simulink model "MultiVehicleModel"  (R2014a)
settings: Solver=ode1  StartTime=0.0  StopTime=inf  FixedStep=simPars.SampleTime  RelTol=1e-3
undefined symbols (not defined in the file or in its folder): DiscIntNeverNeededParam, Earth, Env, eul_0, FWFleet, GVFleet, m, RCFleet, s, WGS84
undefined symbols (not defined in the file): simPars
libraries: simulink x26, aerolibtransform2 x7, instrumentlib x6, Actuator_Lib x5, aerolib6dofsys x4, etargetslib x3, aerolibasang x3, aerolibconvert2 x2, aerolibutil x1, aerolibatmos2 x1, aerolibobsolete x1, aerolibgravity2 x1
(part 2 of 4)

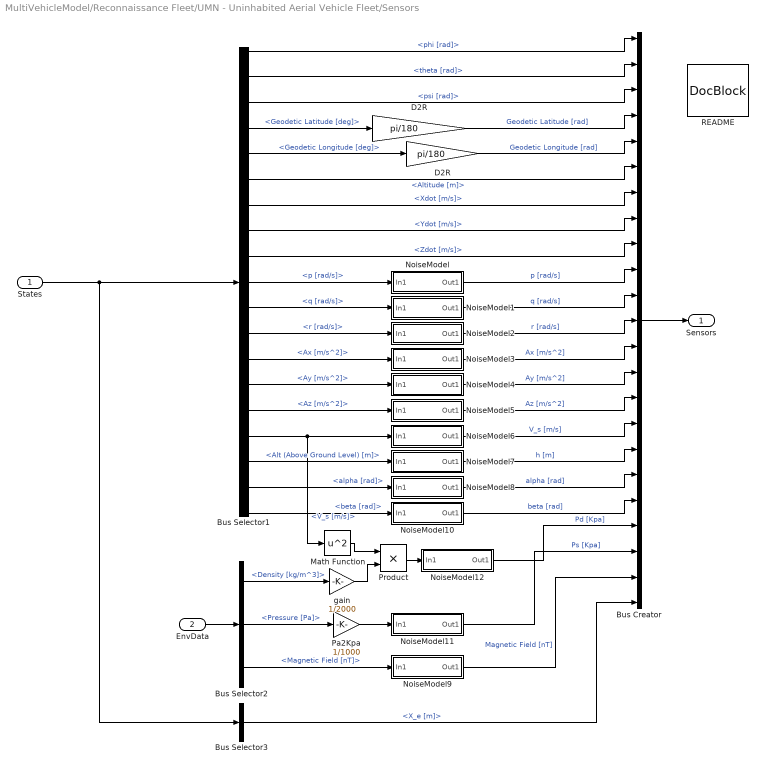
== system MultiVehicleModel/Reconnaissance Fleet/UMN - Uninhabited Aerial Vehicle Fleet/Sensors ==
  States : Inport
  EnvData : Inport  Port=2
  Bus Creator : BusCreator  Inputs=23
  Bus Selector1 : BusSelector  OutputSignals=Euler [rad].phi [rad],Euler [rad].theta [rad],Euler [rad].psi [rad],Nav.Geodetic Latitude [deg],Nav.Geodetic Longitude [deg],Nav.Altitude [m],V_e [m/s].Xdot [m/s],V_e [m/s].Ydot [m/s],V_e [m/s].Zdot [m/s],AngVel [rad/s].p [rad/s],AngVel [rad/s].q [rad/s],AngVel [rad/s].r [rad/s],Accels [m/s^2].Ax [m/s^2],Accels [m/s^2].Ay [m/s^2],Accels [m/s^2].Az [m/s^2],WindAxesParam.V_s [m/s],Nav.Alt (Above Ground Level) [m],WindAxesParam.alpha [rad],WindAxesParam.beta [rad]
  Bus Selector2 : BusSelector  OutputSignals=Density [kg/m^3],Pressure [Pa],Magnetic Field [nT]
  Bus Selector3 : BusSelector  OutputSignals=X_e [m]
  D2R : Gain  Gain=pi/180  SampleTime=SampleTime
  "D2R " : Gain  Gain=pi/180  SampleTime=SampleTime
  Math Function : Math  Operator=square  SaturateOnIntegerOverflow=on
  NoiseModel : Subsystem  mask(Sensor Model){noise_on=AC.Sensors.NoiseOn, sigma=AC.Sensors.IMU.p_noise, seed=878230, bias=AC.Sensors.IMU.p_bias, scf=AC.Sensors.IMU.p_scf, timestep=SampleTime}
      mask prompts: noise_on "on/off"; scf "scale factor:"
      mask help:
      | Add bias, scale factor, and white noise to a signal
      |
      | - 'on/off': 1 = noise on, 0 = noise off.
      | - 'sigma' : Standard deviation of white noise.
      | - 'seed'  : Random number seed.
      | - 'bias'  : Constant mean value offset of white noise.
      | - 'scale factor' : Scale factor applied to original signal.
      | - 'Timestep': Time step of the simulation
      mask Display: disp('bias/scf/noise')
  NoiseModel1 : Subsystem  mask(Sensor Model){noise_on=AC.Sensors.NoiseOn, sigma=AC.Sensors.IMU.q_noise, seed=878231, bias=AC.Sensors.IMU.q_bias, scf=AC.Sensors.IMU.q_scf, timestep=SampleTime}
      mask prompts: noise_on "on/off"; scf "scale factor:"
      mask help:
      | Add bias, scale factor, and white noise to a signal
      |
      | - 'on/off': 1 = noise on, 0 = noise off.
      | - 'sigma' : Standard deviation of white noise.
      | - 'seed'  : Random number seed.
      | - 'bias'  : Constant mean value offset of white noise.
      | - 'scale factor' : Scale factor applied to original signal.
      | - 'Timestep': Time step of the simulation
      mask Display: disp('bias/scf/noise')
  NoiseModel10 : Subsystem  mask(Sensor Model){noise_on=AC.Sensors.NoiseOn, sigma=AC.Sensors.AirData.beta_noise, seed=87828, bias=AC.Sensors.AirData.beta_bias, scf=AC.Sensors.AirData.beta_scf, timestep=SampleTime}
      mask prompts: noise_on "on/off"; scf "scale factor:"
      mask help:
      | Add bias, scale factor, and white noise to a signal
      |
      | - 'on/off': 1 = noise on, 0 = noise off.
      | - 'sigma' : Standard deviation of white noise.
      | - 'seed'  : Random number seed.
      | - 'bias'  : Constant mean value offset of white noise.
      | - 'scale factor' : Scale factor applied to original signal.
      | - 'Timestep': Time step of the simulation
      mask Display: disp('bias/scf/noise')
  NoiseModel11 : Subsystem  mask(Sensor Model){noise_on=AC.Sensors.NoiseOn, sigma=AC.Sensors.AirData.Ps_noise, seed=8782378, bias=AC.Sensors.AirData.Ps_bias, scf=AC.Sensors.AirData.Ps_scf, timestep=SampleTime}
      mask prompts: noise_on "on/off"; scf "scale factor:"
      mask help:
      | Add bias, scale factor, and white noise to a signal
      |
      | - 'on/off': 1 = noise on, 0 = noise off.
      | - 'sigma' : Standard deviation of white noise.
      | - 'seed'  : Random number seed.
      | - 'bias'  : Constant mean value offset of white noise.
      | - 'scale factor' : Scale factor applied to original signal.
      | - 'Timestep': Time step of the simulation
      mask Display: disp('bias/scf/noise')
  NoiseModel12 : Subsystem  mask(Sensor Model){noise_on=AC.Sensors.NoiseOn, sigma=AC.Sensors.AirData.Pd_noise, seed=87823, bias=AC.Sensors.AirData.Pd_bias, scf=AC.Sensors.AirData.Pd_scf, timestep=SampleTime}
      mask prompts: noise_on "on/off"; scf "scale factor:"
      mask help:
      | Add bias, scale factor, and white noise to a signal
      |
      | - 'on/off': 1 = noise on, 0 = noise off.
      | - 'sigma' : Standard deviation of white noise.
      | - 'seed'  : Random number seed.
      | - 'bias'  : Constant mean value offset of white noise.
      | - 'scale factor' : Scale factor applied to original signal.
      | - 'Timestep': Time step of the simulation
      mask Display: disp('bias/scf/noise')
  NoiseModel2 : Subsystem  mask(Sensor Model){noise_on=AC.Sensors.NoiseOn, sigma=AC.Sensors.IMU.r_noise, seed=878232, bias=AC.Sensors.IMU.r_bias, scf=AC.Sensors.IMU.r_scf, timestep=SampleTime}
      mask prompts: noise_on "on/off"; scf "scale factor:"
      mask help:
      | Add bias, scale factor, and white noise to a signal
      |
      | - 'on/off': 1 = noise on, 0 = noise off.
      | - 'sigma' : Standard deviation of white noise.
      | - 'seed'  : Random number seed.
      | - 'bias'  : Constant mean value offset of white noise.
      | - 'scale factor' : Scale factor applied to original signal.
      | - 'Timestep': Time step of the simulation
      mask Display: disp('bias/scf/noise')
  NoiseModel3 : Subsystem  mask(Sensor Model){noise_on=AC.Sensors.NoiseOn, sigma=AC.Sensors.IMU.ax_noise, seed=878233, bias=AC.Sensors.IMU.ax_bias, scf=AC.Sensors.IMU.ax_scf, timestep=SampleTime}
      mask prompts: noise_on "on/off"; scf "scale factor:"
      mask help:
      | Add bias, scale factor, and white noise to a signal
      |
      | - 'on/off': 1 = noise on, 0 = noise off.
      | - 'sigma' : Standard deviation of white noise.
      | - 'seed'  : Random number seed.
      | - 'bias'  : Constant mean value offset of white noise.
      | - 'scale factor' : Scale factor applied to original signal.
      | - 'Timestep': Time step of the simulation
      mask Display: disp('bias/scf/noise')
  NoiseModel4 : Subsystem  mask(Sensor Model){noise_on=AC.Sensors.NoiseOn, sigma=AC.Sensors.IMU.ay_noise, seed=878234, bias=AC.Sensors.IMU.ay_bias, scf=AC.Sensors.IMU.ay_scf, timestep=SampleTime}
      mask prompts: noise_on "on/off"; scf "scale factor:"
      mask help:
      | Add bias, scale factor, and white noise to a signal
      |
      | - 'on/off': 1 = noise on, 0 = noise off.
      | - 'sigma' : Standard deviation of white noise.
      | - 'seed'  : Random number seed.
      | - 'bias'  : Constant mean value offset of white noise.
      | - 'scale factor' : Scale factor applied to original signal.
      | - 'Timestep': Time step of the simulation
      mask Display: disp('bias/scf/noise')
  NoiseModel5 : Subsystem  mask(Sensor Model){noise_on=AC.Sensors.NoiseOn, sigma=AC.Sensors.IMU.az_noise, seed=878235, bias=AC.Sensors.IMU.az_bias, scf=AC.Sensors.IMU.az_scf, timestep=SampleTime}
      mask prompts: noise_on "on/off"; scf "scale factor:"
      mask help:
      | Add bias, scale factor, and white noise to a signal
      |
      | - 'on/off': 1 = noise on, 0 = noise off.
      | - 'sigma' : Standard deviation of white noise.
      | - 'seed'  : Random number seed.
      | - 'bias'  : Constant mean value offset of white noise.
      | - 'scale factor' : Scale factor applied to original signal.
      | - 'Timestep': Time step of the simulation
      mask Display: disp('bias/scf/noise')
  NoiseModel6 : Subsystem  mask(Sensor Model){noise_on=AC.Sensors.NoiseOn, sigma=AC.Sensors.AirData.ias_noise, seed=878236, bias=AC.Sensors.AirData.ias_bias, scf=AC.Sensors.AirData.ias_scf, timestep=SampleTime}
      mask prompts: noise_on "on/off"; scf "scale factor:"
      mask help:
      | Add bias, scale factor, and white noise to a signal
      |
      | - 'on/off': 1 = noise on, 0 = noise off.
      | - 'sigma' : Standard deviation of white noise.
      | - 'seed'  : Random number seed.
      | - 'bias'  : Constant mean value offset of white noise.
      | - 'scale factor' : Scale factor applied to original signal.
      | - 'Timestep': Time step of the simulation
      mask Display: disp('bias/scf/noise')
  NoiseModel7 : Subsystem  mask(Sensor Model){noise_on=AC.Sensors.NoiseOn, sigma=AC.Sensors.AirData.h_noise, seed=87828, bias=AC.Sensors.AirData.h_bias, scf=AC.Sensors.AirData.h_scf, timestep=SampleTime}
      mask prompts: noise_on "on/off"; scf "scale factor:"
      mask help:
      | Add bias, scale factor, and white noise to a signal
      |
      | - 'on/off': 1 = noise on, 0 = noise off.
      | - 'sigma' : Standard deviation of white noise.
      | - 'seed'  : Random number seed.
      | - 'bias'  : Constant mean value offset of white noise.
      | - 'scale factor' : Scale factor applied to original signal.
      | - 'Timestep': Time step of the simulation
      mask Display: disp('bias/scf/noise')
  NoiseModel8 : Subsystem  mask(Sensor Model){noise_on=AC.Sensors.NoiseOn, sigma=AC.Sensors.AirData.alpha_noise, seed=87828, bias=AC.Sensors.AirData.alpha_bias, scf=AC.Sensors.AirData.alpha_scf, timestep=SampleTime}
      mask prompts: noise_on "on/off"; scf "scale factor:"
      mask help:
      | Add bias, scale factor, and white noise to a signal
      |
      | - 'on/off': 1 = noise on, 0 = noise off.
      | - 'sigma' : Standard deviation of white noise.
      | - 'seed'  : Random number seed.
      | - 'bias'  : Constant mean value offset of white noise.
      | - 'scale factor' : Scale factor applied to original signal.
      | - 'Timestep': Time step of the simulation
      mask Display: disp('bias/scf/noise')
  NoiseModel9 : Subsystem  mask(Sensor Model){noise_on=AC.Sensors.NoiseOn, sigma=[AC.Sensors.IMU.hx_noise, AC.Sensors.IMU.hy_noise,AC.Sensors.IMU.hz_noise], seed=878237, bias=[AC.Sensors.IMU.hx_bias, AC.Sensors.IMU.hy_bias, AC.Sensors.IMU.hz_bias], scf=[AC.Sensors.IMU.hx_scf, AC.Sensors.IMU.hy_scf, AC.Sensors.IMU.hz_scf], timestep=SampleTime}
      mask prompts: noise_on "on/off"; scf "scale factor:"
      mask help:
      | Add bias, scale factor, and white noise to a signal
      |
      | - 'on/off': 1 = noise on, 0 = noise off.
      | - 'sigma' : Standard deviation of white noise.
      | - 'seed'  : Random number seed.
      | - 'bias'  : Constant mean value offset of white noise.
      | - 'scale factor' : Scale factor applied to original signal.
      | - 'Timestep': Time step of the simulation
      mask Display: disp('bias/scf/noise')
  Pa2Kpa : Gain  Gain=1/1000
  Product : Product  RndMeth=Zero
  README : simulink/Model-Wide Utilities/DocBlock  DocumentType=Text
      content=|
      | Sensors
      |
      | This block implements sensor models on selected signals. A generic block
      | is used that applies a bias, scale factor, and band limited white noise to
      | a given signal. The parameters for each block are stored in the aircraft
      | configuration data structure (AC):
      |
      | >> AC.Sensors
      |
      | ans =
      |
      |     NoiseOn: 1
      |         IMU: [1x1 struct]
      |     AirData: [1x1 struct]
      |
      | Note the "NoiseOn" boolean flag- by setting this flag to zero, the sensor
      | model will be disabled.
      |
      | Currently, the bias and scale factor errors are not used; only white noise
      | is applied.
  gain : Gain  Gain=1/2000
  Sensors : Outport
  wires:
  Bus Selector1/15 -> NoiseModel5/1(In1)  "<Az [m/s^2]>"
  Bus Selector1/14 -> NoiseModel4/1(In1)  "<Ay [m/s^2]>"
  Bus Selector1/13 -> NoiseModel3/1(In1)  "<Ax [m/s^2]>"
  Bus Selector1/12 -> NoiseModel2/1(In1)  "<r [rad/s]>"
  Bus Selector1/11 -> NoiseModel1/1(In1)  "<q [rad/s]>"
  Bus Selector1/10 -> NoiseModel/1(In1)  "<p [rad/s]>"
  States/1 -> Bus Selector3/1, Bus Selector1/1
  Bus Selector1/16 -> NoiseModel6/1(In1), Math Function/1  "<V_s [m/s]>"
  Bus Selector2/3 -> NoiseModel9/1(In1)  "<Magnetic Field [nT]>"
  Bus Selector1/17 -> NoiseModel7/1(In1)  "<Alt (Above Ground Level) [m]>"
  EnvData/1 -> Bus Selector2/1
  Bus Selector1/18 -> NoiseModel8/1(In1)  "<alpha [rad]>"
  Bus Selector1/19 -> NoiseModel10/1(In1)  "<beta [rad]>"
  Bus Selector2/2 -> Pa2Kpa/1  "<Pressure [Pa]>"
  Pa2Kpa/1 -> NoiseModel11/1(In1)
  Bus Selector2/1 -> gain/1  "<Density [kg/m^3]>"
  Math Function/1 -> Product/1
  gain/1 -> Product/2
  Product/1 -> NoiseModel12/1(In1)
  Bus Creator/1 -> Sensors/1
  Bus Selector1/1 -> Bus Creator/1  "<phi [rad]>"
  Bus Selector1/2 -> Bus Creator/2  "<theta [rad]>"
  Bus Selector1/3 -> Bus Creator/3  "<psi [rad]>"
  Bus Selector1/4 -> D2R/1  "<Geodetic Latitude [deg]>"
  Bus Selector1/5 -> "D2R "/1  "<Geodetic Longitude [deg]>"
  Bus Selector1/6 -> Bus Creator/6  "<Altitude [m]>"
  Bus Selector1/7 -> Bus Creator/7  "<Xdot [m/s]>"
  Bus Selector1/8 -> Bus Creator/8  "<Ydot [m/s]>"
  Bus Selector1/9 -> Bus Creator/9  "<Zdot [m/s]>"
  NoiseModel/1(Out1) -> Bus Creator/10  "p [rad/s]"
  NoiseModel1/1(Out1) -> Bus Creator/11  "q [rad/s]"
  NoiseModel2/1(Out1) -> Bus Creator/12  "r [rad/s]"
  NoiseModel3/1(Out1) -> Bus Creator/13  "Ax [m/s^2]"
  NoiseModel4/1(Out1) -> Bus Creator/14  "Ay [m/s^2]"
  NoiseModel5/1(Out1) -> Bus Creator/15  "Az [m/s^2]"
  NoiseModel6/1(Out1) -> Bus Creator/16  "V_s [m/s]"
  NoiseModel7/1(Out1) -> Bus Creator/17  "h [m]"
  NoiseModel8/1(Out1) -> Bus Creator/18  "alpha [rad]"
  NoiseModel10/1(Out1) -> Bus Creator/19  "beta [rad]"
  NoiseModel12/1(Out1) -> Bus Creator/20  "Pd [Kpa]"
  NoiseModel11/1(Out1) -> Bus Creator/21  "Ps [Kpa]"
  NoiseModel9/1(Out1) -> Bus Creator/22  "Magnetic Field [nT]"
  D2R/1 -> Bus Creator/4  "Geodetic Latitude [rad]"
  "D2R "/1 -> Bus Creator/5  "Geodetic Longitude [rad]"
  Bus Selector3/1 -> Bus Creator/23  "<X_e [m]>"

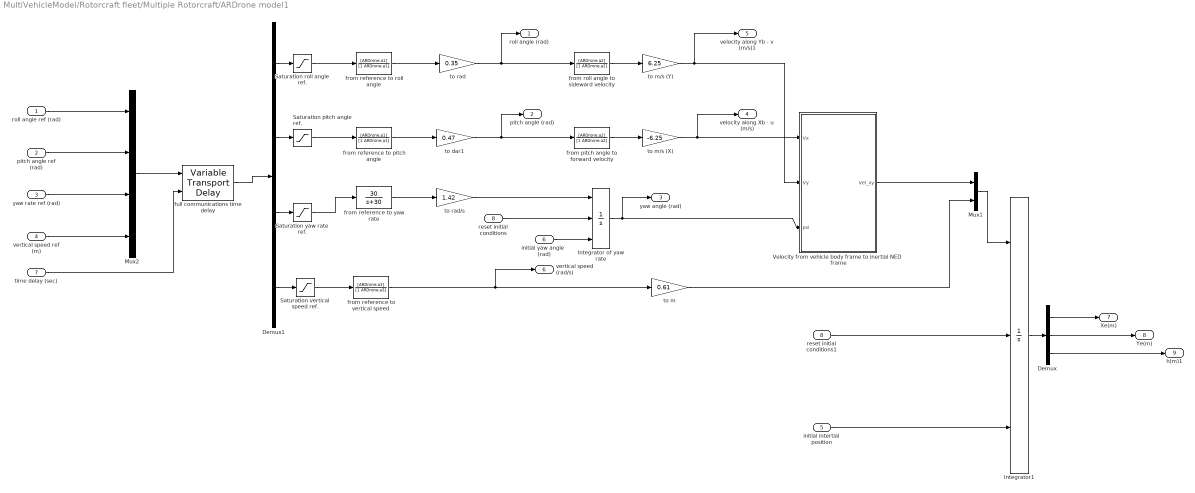
== system MultiVehicleModel/Rotorcraft fleet/Multiple Rotorcraft/ARDrone model1 ==
  roll angle ref (rad) : Inport
  pitch angle ref (rad) : Inport  Port=2
  yaw rate ref (rad) : Inport  Port=3
  vertical speed ref (m) : Inport  Port=4
  initial intertial position : Inport  Port=5
  initial yaw angle  (rad) : Inport  Port=6
  time delay (sec) : Inport  Port=7
  reset initial conditions : Inport  Port=8
  Demux : Demux  Outputs=3
  Demux1 : Demux
  Integrator of yaw rate : Integrator  ExternalReset=rising  InitialConditionSource=external
  Integrator1 : Integrator  ExternalReset=rising  InitialConditionSource=external
  Mux1 : Mux  Inputs=2
  Mux2 : Mux
  Saturation pitch angle ref. : Saturate  UpperLimit=ARDrone.MAX_ANGLE_REF  LowerLimit=ARDrone.MIN_ANGLE_REF
  Saturation roll angle ref. : Saturate  UpperLimit=ARDrone.MAX_ANGLE_REF  LowerLimit=ARDrone.MIN_ANGLE_REF
  Saturation vertical speed ref. : Saturate  UpperLimit=ARDrone.MAX_VERTICAL_SPEED  LowerLimit=ARDrone.MIN_VERTICAL_SPEED
  Saturation yaw rate ref. : Saturate  UpperLimit=ARDrone.MAX_YAW_RATE_REF  LowerLimit=ARDrone.MIN_YAW_RATE_REF
  Velocity from vehicle body frame to inertial NED  frame : MATLAB Function  TreatAsAtomicUnit=on
  from pitch angle to forward velocity : TransferFcn  Numerator=[ARDrone.a2]  Denominator=[1 ARDrone.a2]
  from reference to pitch angle : TransferFcn  Numerator=[ARDrone.a1]  Denominator=[1 ARDrone.a1]
  from reference to roll angle : TransferFcn  Numerator=[ARDrone.a1]  Denominator=[1 ARDrone.a1]
  from reference to vertical speed : TransferFcn  Numerator=[ARDrone.a3]  Denominator=[1 ARDrone.a3]
  from reference to yaw rate : TransferFcn  Numerator=[30]  Denominator=[1 30]
  from roll angle to sideward velocity : TransferFcn  Numerator=[ARDrone.a2]  Denominator=[1 ARDrone.a2]
  full communications time delay : VariableTransportDelay  MaximumDelay=10  InitialOutput=[0 0 0 0]
  reset initial conditions1 : InportShadow  Port=8
  to dar1 : Gain  Gain=0.47
  to m : Gain  Gain=0.61
  to m/s (X) : Gain  Gain=-6.25
  to m/s (Y) : Gain  Gain=6.25
  to rad : Gain  Gain=0.35
  to rad/s : Gain  Gain=1.42
  roll angle (rad) : Outport
  pitch angle (rad) : Outport  Port=2
  yaw angle (rad) : Outport  Port=3
  velocity along Xb - u (m/s) : Outport  Port=4
  velocity along Yb - v (m/s)1 : Outport  Port=5
  vertical speed (rad/s) : Outport  Port=6
  Xe(m) : Outport  Port=7
  Ye(m) : Outport  Port=8
  h(m)1 : Outport  Port=9
  wires:
  from reference to pitch angle/1 -> to dar1/1
  from reference to roll angle/1 -> to rad/1
  Saturation roll angle ref./1 -> from reference to roll angle/1
  from reference to yaw rate/1 -> to rad/s/1
  Saturation vertical speed ref./1 -> from reference to vertical speed/1
  from pitch angle to forward velocity/1 -> to m/s (X)/1
  from roll angle to sideward velocity/1 -> to m/s (Y)/1
  Demux1/2 -> Saturation pitch angle ref./1
  Demux1/3 -> Saturation yaw rate ref./1
  Integrator of yaw rate/1 -> Velocity from vehicle body frame to inertial NED  frame/3(psi), yaw angle (rad)/1
  Mux1/1 -> Integrator1/1
  Velocity from vehicle body frame to inertial NED  frame/1(Vel_xy) -> Mux1/1
  from reference to vertical speed/1 -> vertical speed (rad/s)/1, to m/1
  Integrator1/1 -> Demux/1
  Demux1/1 -> Saturation roll angle ref./1
  to rad/1 -> from roll angle to sideward velocity/1, roll angle (rad)/1
  to dar1/1 -> from pitch angle to forward velocity/1, pitch angle (rad)/1
  Demux/3 -> h(m)1/1
  Demux/2 -> Ye(m)/1
  Demux/1 -> Xe(m)/1
  time delay (sec)/1 -> full communications time delay/2
  Mux2/1 -> full communications time delay/1
  full communications time delay/1 -> Demux1/1
  roll angle ref (rad)/1 -> Mux2/1
  pitch angle ref (rad)/1 -> Mux2/2
  yaw rate ref (rad)/1 -> Mux2/3
  vertical speed ref (m)/1 -> Mux2/4
  Demux1/4 -> Saturation vertical speed ref./1
  initial intertial position/1 -> Integrator1/3
  initial yaw angle  (rad)/1 -> Integrator of yaw rate/3
  reset initial conditions/1 -> Integrator of yaw rate/2
  reset initial conditions1/1 -> Integrator1/2
  to rad/s/1 -> Integrator of yaw rate/1
  to m/s (X)/1 -> Velocity from vehicle body frame to inertial NED  frame/1(Vx), velocity along Xb - u (m/s)/1
  to m/1 -> Mux1/2
  Saturation yaw rate ref./1 -> from reference to yaw rate/1
  to m/s (Y)/1 -> Velocity from vehicle body frame to inertial NED  frame/2(Vy), velocity along Yb - v (m/s)1/1
  Saturation pitch angle ref./1 -> from reference to pitch angle/1

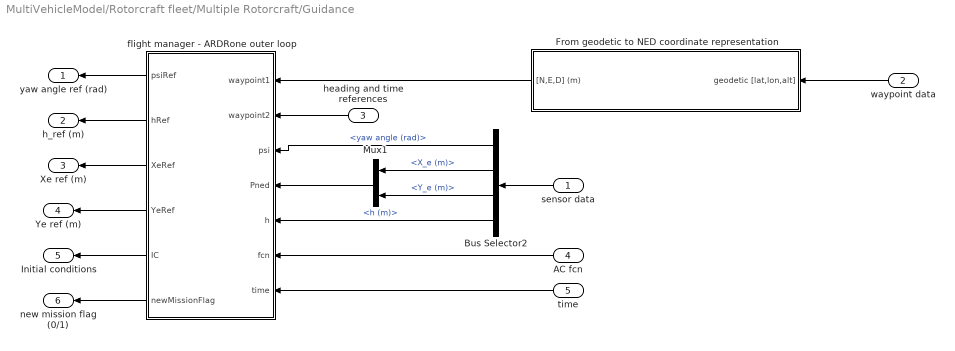
== system MultiVehicleModel/Rotorcraft fleet/Multiple Rotorcraft/Guidance  ==
  sensor data : Inport
  waypoint data : Inport  Port=2
  heading and time references : Inport  Port=3
  AC fcn : Inport  Port=4
  time : Inport  Port=5
  Bus Selector2 : BusSelector  OutputSignals=yaw angle (rad),X_e (m),Y_e (m),h (m)
  From geodetic to NED coordinate representation : Subsystem  TreatAsAtomicUnit=on
  Mux1 : Mux  Inputs=2
  flight manager - ARDRone outer loop : MATLAB Function  TreatAsAtomicUnit=on
  yaw angle ref (rad) : Outport
  h_ref (m) : Outport  Port=2
  Xe ref (m) : Outport  Port=3
  Ye ref (m) : Outport  Port=4
  Initial conditions : Outport  Port=5
  new mission flag (0/1) : Outport  Port=6
  wires:
  Bus Selector2/2 -> Mux1/1  "<X_e (m)>"
  Bus Selector2/3 -> Mux1/2  "<Y_e (m)>"
  sensor data/1 -> Bus Selector2/1
  Bus Selector2/1 -> flight manager - ARDRone outer loop/3(psi)  "<yaw angle (rad)>"
  Mux1/1 -> flight manager - ARDRone outer loop/4(Pned)
  waypoint data/1 -> From geodetic to NED coordinate representation/1(geodetic [lat,lon,alt])
  AC fcn/1 -> flight manager - ARDRone outer loop/6(fcn)
  flight manager - ARDRone outer loop/2(hRef) -> h_ref (m)/1
  flight manager - ARDRone outer loop/1(psiRef) -> yaw angle ref (rad)/1
  flight manager - ARDRone outer loop/3(XeRef) -> Xe ref (m)/1
  flight manager - ARDRone outer loop/4(YeRef) -> Ye ref (m)/1
  Bus Selector2/4 -> flight manager - ARDRone outer loop/5(h)  "<h (m)>"
  time/1 -> flight manager - ARDRone outer loop/7(time)
  From geodetic to NED coordinate representation/1("[N,E,D] (m)") -> flight manager - ARDRone outer loop/1(waypoint1)
  heading and time references/1 -> flight manager - ARDRone outer loop/2(waypoint2)
  flight manager - ARDRone outer loop/5(IC) -> Initial conditions/1
  flight manager - ARDRone outer loop/6(newMissionFlag) -> new mission flag (0/1)/1

== system MultiVehicleModel/Rotorcraft fleet/Multiple Rotorcraft/Navigation ==
  X_e [m] : Inport
  Bus Creator1 : BusCreator  Inputs=6
  Demux : Demux  Outputs=2
  EGM-96 Geoid Model : Subsystem  mask(EGM-96 geoid undulation model){}
      mask help: Computes the MSL (mean sea level) altitude as a function of position.
      mask init:
      | load('egm96');
      mask Help:
      | The block computes the mean-sea-level altitude relative to the WGS-84 geoid.
      | <P><B>Inputs:</B>
      | <LI>Position = the 3x1 vector of aircraft location [Latitude Longitude Altitude], in [rad rad m]</LI>
      | </P>
      | <P><B>Output:</B>
      | <LI>MSLAlt = the mean-sea-level altitude, in m</LI>
      | </P>
  Flat Earth to LLA : aerolibtransform2/Flat Earth to LLA  units=Metric (MKS)  ptype=Earth (WGS84)  F=1/298.257223563  R=6378137  LL0=RCFleet.IC.geodetic(1:2)  psi=0
  Ground Detection : Subsystem  mask(Ground detection){}
      mask help: Computes altitude above ground and sets a flag if AGL is negative.
      mask Help:
      | The block computes the altitude above ground (AGL) and sets a flag if the AGL is negative (used for ground contact detection).
      | <P><B>Inputs:</B>
      | <LI>MSLAlt = the altitude measured from mean-sea-level, in meters</LI>
      | <LI>GndAlt = the altitude of the terrain (above MSL) at current location, in meters</LI>
      | </P>
      | <P><B>Output:</B>
      | <LI>AConGnd = the aircraft-on-ground flag (0 if aircraft above ground, 1 if aircraft on the ground)</LI>
      | <LI>AGLAlt = the altitude of the aircraft above ground</LI>
      | </P>
  Ground Height : Constant  Value=Env.GroundAlt
  Ground Height1 : Constant  Value=Env.GroundAlt
  Latitude Bound [-180,180] : Subsystem
  Longitude Bound 0-360 : Subsystem  mask(Longitude bound){}
      mask help: Bounds the longitude to [0, 2pi]. When 0 bound is exceeded the longitude wraps back to 2pi; when the 2pi bound is exceeded the longitude wraps back to 0.
  Mux : Mux  Inputs=3
  README : simulink/Model-Wide Utilities/DocBlock  DocumentType=Text
      content=|
      | Navigation
      |
      | This block is library link that contains the navigational model and
      | equations. Included are equations relating the flat Earth position to
      | latitude/longitude, a simplified 2D table lookup version of the EGM-96
      | Geoid model for computation of MSL/AGL altitudes, and computation of
      | flight path and ground track angles.
  Saturation : Saturate  UpperLimit=Inf  LowerLimit=0
  Nav : Outport
  wires:
  Ground Detection/2(AGLAlt) -> Bus Creator1/6  "Alt (Above Ground Level) [m]"
  Saturation/1 -> Mux/3, Bus Creator1/3  "Altitude [m]"
  Ground Detection/1(AConGnd) -> Bus Creator1/5  "AC on Ground"
  Ground Height1/1 -> Ground Detection/2(GndAlt)
  EGM-96 Geoid Model/1(MSLAlt) -> Bus Creator1/4, Ground Detection/1(MSLAlt)  "Alt (Above Mean Sea Level) [m]"
  Bus Creator1/1 -> Nav/1
  Ground Height/1 -> Flat Earth to LLA/2
  X_e [m]/1 -> Flat Earth to LLA/1
  Demux/2 -> Longitude Bound 0-360/1(In), Bus Creator1/2  "Geodetic Longitude [deg]"
  Demux/1 -> Bus Creator1/1, Latitude Bound [-180,180]/1(In)  "Geodetic Latitude [deg]"
  Flat Earth to LLA/2 -> Saturation/1  "Altitude [m]"
  Flat Earth to LLA/1 -> Demux/1
  Mux/1 -> EGM-96 Geoid Model/1(Position)
  Longitude Bound 0-360/1(Out) -> Mux/2
  Latitude Bound [-180,180]/1(Out) -> Mux/1

== system MultiVehicleModel/Rotorcraft fleet/Multiple Rotorcraft/data to send ==
  nav data : Inport
  heading angle (rad) : Inport  Port=2
  pitch angle (rad) : Inport  Port=3
  roll angle (rad) : Inport  Port=4
  Bus Selector : BusSelector  OutputSignals=Geodetic Latitude [deg],Geodetic Longitude [deg],Altitude [m]
  Gain1 : Gain  Gain=180/pi
  Gain2 : Gain  Gain=-180/pi
  Gain3 : Gain  Gain=-180/pi
  Mux : Mux  Inputs=6
  data out : Outport
  wires:
  Gain1/1 -> Mux/4
  Bus Selector/3 -> Mux/3  "<Altitude [m]>"
  Mux/1 -> data out/1
  nav data/1 -> Bus Selector/1
  Bus Selector/1 -> Mux/1  "<Geodetic Latitude [deg]>"
  Bus Selector/2 -> Mux/2  "<Geodetic Longitude [deg]>"
  heading angle (rad)/1 -> Gain1/1
  pitch angle (rad)/1 -> Gain2/1
  Gain2/1 -> Mux/5
  roll angle (rad)/1 -> Gain3/1
  Gain3/1 -> Mux/6

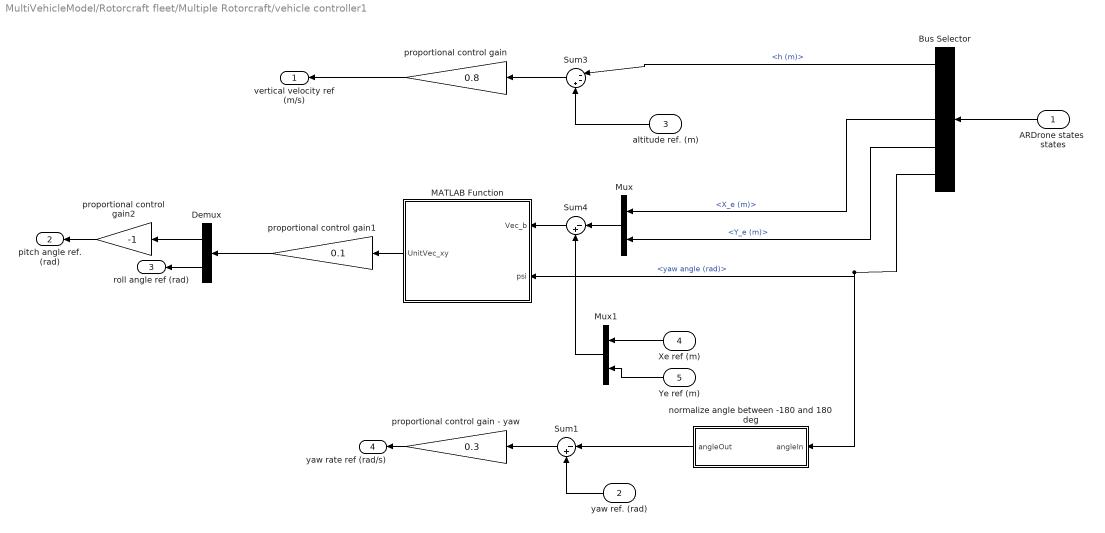
== system MultiVehicleModel/Rotorcraft fleet/Multiple Rotorcraft/vehicle controller1 ==
  "ARDrone states  states " : Inport
  yaw ref. (rad) : Inport  Port=2
  altitude ref. (m) : Inport  Port=3
  Xe ref (m) : Inport  Port=4
  Ye ref (m) : Inport  Port=5
  Bus Selector : BusSelector  OutputSignals=h (m),vertical velocity - h_dot (m/s),X_e (m),Y_e (m),yaw angle (rad)
  Demux : Demux  Outputs=2
  MATLAB Function : MATLAB Function  TreatAsAtomicUnit=on
  Mux : Mux  Inputs=2
  Mux1 : Mux  Inputs=2
  Sum1 : Sum  Inputs=|-+
  Sum3 : Sum  Inputs=|--+
  Sum4 : Sum  Inputs=|-+
  normalize angle between -180 and 180 deg : MATLAB Function  TreatAsAtomicUnit=on
  proportional control gain : Gain  Gain=0.8
  proportional control gain - yaw : Gain  Gain=0.3
  proportional control gain1 : Gain  Gain=0.1
  proportional control gain2 : Gain  Gain=-1
  vertical velocity ref (m/s) : Outport
  pitch angle ref. (rad) : Outport  Port=2
  roll angle ref (rad) : Outport  Port=3
  yaw rate ref (rad/s) : Outport  Port=4
  wires:
  proportional control gain - yaw/1 -> yaw rate ref (rad/s)/1
  Demux/1 -> proportional control gain2/1
  proportional control gain/1 -> vertical velocity ref (m/s)/1
  Demux/2 -> roll angle ref (rad)/1
  proportional control gain1/1 -> Demux/1
  Mux1/1 -> Sum4/2
  Sum4/1 -> MATLAB Function/1(Vec_b)
  Bus Selector/4 -> Mux/2  "<Y_e (m)>"
  MATLAB Function/1(UnitVec_xy) -> proportional control gain1/1
  Sum3/1 -> proportional control gain/1
  Bus Selector/1 -> Sum3/1  "<h (m)>"
  Bus Selector/3 -> Mux/1  "<X_e (m)>"
  Bus Selector/5 -> normalize angle between -180 and 180 deg/1(angleIn), MATLAB Function/2(psi)  "<yaw angle (rad)>"
  Mux/1 -> Sum4/1
  altitude ref. (m)/1 -> Sum3/3
  normalize angle between -180 and 180 deg/1(angleOut) -> Sum1/1
  Sum1/1 -> proportional control gain - yaw/1
  "ARDrone states  states "/1 -> Bus Selector/1
  Xe ref (m)/1 -> Mux1/1
  Ye ref (m)/1 -> Mux1/2
  yaw ref. (rad)/1 -> Sum1/2
  proportional control gain2/1 -> pitch angle ref. (rad)/1

== system MultiVehicleModel/Ground Vehicle fleet/Model of ground vehicle fleet/Guidance algorithm/From geodetic to NED coordinate representation ==
  geodetic [lat,lon,alt] : Inport  Partition=on  PartitionDimension=2  PartitionWidth=1
  Demux : Demux  Outputs=[2 1]
  For Each : ForEach  DisableCoverage=on  IndexMode=One-based
  Ground Height1 : Constant  Value=Env.GroundAlt
  LLA to Flat Earth : aerolibtransform2/LLA to Flat Earth  units=Metric (MKS)  ptype=Earth (WGS84)  F=1/298.257223563  R=6378137  LL0=FWFleet.IC.geodetic(1:2)  psi=0
  "[N,E,D] (m)" : Outport  ConcatenationDimension=2
  wires:
  LLA to Flat Earth/1 -> "[N,E,D] (m)"/1
  Demux/1 -> LLA to Flat Earth/1
  Demux/2 -> LLA to Flat Earth/2
  geodetic [lat,lon,alt]/1 -> Demux/1
  Ground Height1/1 -> LLA to Flat Earth/3

== system MultiVehicleModel/Ground Vehicle fleet/Model of ground vehicle fleet/Navigation/EGM-96 Geoid Model ==
  Position : Inport
  Demux2 : Demux  Outputs=3
  Look-Up Table (2-D) : Lookup2D  RowIndex=Lat  ColumnIndex=Lon  Table=Alterr'  SaturateOnIntegerOverflow=on  InputSameDT=on
  Sum : Sum  Inputs=|+++
  WGS-84 correction : Constant  Value=-0.53
  MSLAlt : Outport
  wires:
  Demux2/2 -> Look-Up Table (2-D)/2
  Demux2/1 -> Look-Up Table (2-D)/1
  Position/1 -> Demux2/1
  Demux2/3 -> Sum/2
  Sum/1 -> MSLAlt/1
  Look-Up Table (2-D)/1 -> Sum/1
  WGS-84 correction/1 -> Sum/3

== system MultiVehicleModel/Ground Vehicle fleet/Model of ground vehicle fleet/Navigation/Ground Detection ==
  MSLAlt : Inport
  GndAlt : Inport  Port=2
  False : Constant  Value=0
  Sum : Sum  Inputs=|+-  SaturateOnIntegerOverflow=on  InputSameDT=on  OutDataTypeStr=Inherit: Same as first input
  Switch : Switch  SaturateOnIntegerOverflow=on  InputSameDT=on
  True : Constant
  AConGnd : Outport
  AGLAlt : Outport  Port=2
  wires:
  MSLAlt/1 -> Sum/1
  GndAlt/1 -> Sum/2
  Sum/1 -> Switch/2, AGLAlt/1
  False/1 -> Switch/1
  True/1 -> Switch/3
  Switch/1 -> AConGnd/1

== system MultiVehicleModel/Ground Vehicle fleet/Model of ground vehicle fleet/Navigation/Latitude Bound [-180,180] ==
  In : Inport
  2pi : Constant  Value=360
  Math Function : Math  Operator=mod  SaturateOnIntegerOverflow=on
  Sum1 : Sum  Inputs=|+-  SaturateOnIntegerOverflow=on  InputSameDT=on  OutDataTypeStr=Inherit: Same as first input
  Sum2 : Sum  Inputs=|++  SaturateOnIntegerOverflow=on  InputSameDT=on  OutDataTypeStr=Inherit: Same as first input
  pi : Constant  Value=180
  Out : Outport
  wires:
  Math Function/1 -> Sum1/1
  2pi/1 -> Math Function/2
  In/1 -> Sum2/1
  Sum2/1 -> Math Function/1
  pi/1 -> Sum2/2, Sum1/2
  Sum1/1 -> Out/1

== system MultiVehicleModel/Ground Vehicle fleet/Model of ground vehicle fleet/Navigation/Longitude Bound 0-360 ==
  In : Inport
  2pi : Constant  Value=360
  Math Function : Math  Operator=mod  SaturateOnIntegerOverflow=on
  Out : Outport
  wires:
  Math Function/1 -> Out/1
  2pi/1 -> Math Function/2
  In/1 -> Math Function/1

== system MultiVehicleModel/Reconnaissance Fleet/UMN - Uninhabited Aerial Vehicle Fleet/Actuators/Elevator Servo ==
  In : Inport
  Gain : Gain  Gain=2*pi*freq  SaturateOnIntegerOverflow=on  OutDataTypeStr=Inherit: Same as input  ParamDataTypeStr=Inherit: Same as input
  Integrator : Integrator  InitialConditionSource=external  LimitOutput=on  UpperSaturationLimit=POS_hi  LowerSaturationLimit=POS_lo  IgnoreLimit=on
  Rate Limiter : Saturate  UpperLimit=RL  LowerLimit=-RL
  Sum : Sum  Inputs=-+|  SaturateOnIntegerOverflow=on  InputSameDT=on  OutDataTypeStr=Inherit: Same as first input
  Out : Outport  PortDimensions=1
  wires:
  In/1 -> Sum/2, Integrator/2
  Rate Limiter/1 -> Integrator/1  "Ydot_lim"
  Integrator/1 -> Out/1, Sum/1  "Y"
  Sum/1 -> Gain/1  "Error"
  Gain/1 -> Rate Limiter/1  "Ydot"

== system MultiVehicleModel/Reconnaissance Fleet/UMN - Uninhabited Aerial Vehicle Fleet/Actuators/Left Aileron Servo ==
  In : Inport
  Gain : Gain  Gain=2*pi*freq  SaturateOnIntegerOverflow=on  OutDataTypeStr=Inherit: Same as input  ParamDataTypeStr=Inherit: Same as input
  Integrator : Integrator  InitialConditionSource=external  LimitOutput=on  UpperSaturationLimit=POS_hi  LowerSaturationLimit=POS_lo  IgnoreLimit=on
  Rate Limiter : Saturate  UpperLimit=RL  LowerLimit=-RL
  Sum : Sum  Inputs=-+|  SaturateOnIntegerOverflow=on  InputSameDT=on  OutDataTypeStr=Inherit: Same as first input
  Out : Outport  PortDimensions=1
  wires:
  In/1 -> Sum/2, Integrator/2
  Rate Limiter/1 -> Integrator/1  "Ydot_lim"
  Integrator/1 -> Out/1, Sum/1  "Y"
  Sum/1 -> Gain/1  "Error"
  Gain/1 -> Rate Limiter/1  "Ydot"

== system MultiVehicleModel/Reconnaissance Fleet/UMN - Uninhabited Aerial Vehicle Fleet/Actuators/Left Flap Servo ==
  In : Inport
  Gain : Gain  Gain=2*pi*freq  SaturateOnIntegerOverflow=on  OutDataTypeStr=Inherit: Same as input  ParamDataTypeStr=Inherit: Same as input
  Integrator : Integrator  InitialConditionSource=external  LimitOutput=on  UpperSaturationLimit=POS_hi  LowerSaturationLimit=POS_lo  IgnoreLimit=on
  Rate Limiter : Saturate  UpperLimit=RL  LowerLimit=-RL
  Sum : Sum  Inputs=-+|  SaturateOnIntegerOverflow=on  InputSameDT=on  OutDataTypeStr=Inherit: Same as first input
  Out : Outport  PortDimensions=1
  wires:
  In/1 -> Sum/2, Integrator/2
  Rate Limiter/1 -> Integrator/1  "Ydot_lim"
  Integrator/1 -> Out/1, Sum/1  "Y"
  Sum/1 -> Gain/1  "Error"
  Gain/1 -> Rate Limiter/1  "Ydot"

== system MultiVehicleModel/Reconnaissance Fleet/UMN - Uninhabited Aerial Vehicle Fleet/Actuators/Right Aileron Servo ==
  In : Inport
  Gain : Gain  Gain=2*pi*freq  SaturateOnIntegerOverflow=on  OutDataTypeStr=Inherit: Same as input  ParamDataTypeStr=Inherit: Same as input
  Integrator : Integrator  InitialConditionSource=external  LimitOutput=on  UpperSaturationLimit=POS_hi  LowerSaturationLimit=POS_lo  IgnoreLimit=on
  Rate Limiter : Saturate  UpperLimit=RL  LowerLimit=-RL
  Sum : Sum  Inputs=-+|  SaturateOnIntegerOverflow=on  InputSameDT=on  OutDataTypeStr=Inherit: Same as first input
  Out : Outport  PortDimensions=1
  wires:
  In/1 -> Sum/2, Integrator/2
  Rate Limiter/1 -> Integrator/1  "Ydot_lim"
  Integrator/1 -> Out/1, Sum/1  "Y"
  Sum/1 -> Gain/1  "Error"
  Gain/1 -> Rate Limiter/1  "Ydot"

== system MultiVehicleModel/Reconnaissance Fleet/UMN - Uninhabited Aerial Vehicle Fleet/Actuators/Right Flap Servo ==
  In : Inport
  Gain : Gain  Gain=2*pi*freq  SaturateOnIntegerOverflow=on  OutDataTypeStr=Inherit: Same as input  ParamDataTypeStr=Inherit: Same as input
  Integrator : Integrator  InitialConditionSource=external  LimitOutput=on  UpperSaturationLimit=POS_hi  LowerSaturationLimit=POS_lo  IgnoreLimit=on
  Rate Limiter : Saturate  UpperLimit=RL  LowerLimit=-RL
  Sum : Sum  Inputs=-+|  SaturateOnIntegerOverflow=on  InputSameDT=on  OutDataTypeStr=Inherit: Same as first input
  Out : Outport  PortDimensions=1
  wires:
  In/1 -> Sum/2, Integrator/2
  Rate Limiter/1 -> Integrator/1  "Ydot_lim"
  Integrator/1 -> Out/1, Sum/1  "Y"
  Sum/1 -> Gain/1  "Error"
  Gain/1 -> Rate Limiter/1  "Ydot"

== system MultiVehicleModel/Reconnaissance Fleet/UMN - Uninhabited Aerial Vehicle Fleet/Actuators/Rudder Servo ==
  In : Inport
  Gain : Gain  Gain=2*pi*freq  SaturateOnIntegerOverflow=on  OutDataTypeStr=Inherit: Same as input  ParamDataTypeStr=Inherit: Same as input
  Integrator : Integrator  InitialConditionSource=external  LimitOutput=on  UpperSaturationLimit=POS_hi  LowerSaturationLimit=POS_lo  IgnoreLimit=on
  Rate Limiter : Saturate  UpperLimit=RL  LowerLimit=-RL
  Sum : Sum  Inputs=-+|  SaturateOnIntegerOverflow=on  InputSameDT=on  OutDataTypeStr=Inherit: Same as first input
  Out : Outport  PortDimensions=1
  wires:
  In/1 -> Sum/2, Integrator/2
  Rate Limiter/1 -> Integrator/1  "Ydot_lim"
  Integrator/1 -> Out/1, Sum/1  "Y"
  Sum/1 -> Gain/1  "Error"
  Gain/1 -> Rate Limiter/1  "Ydot"

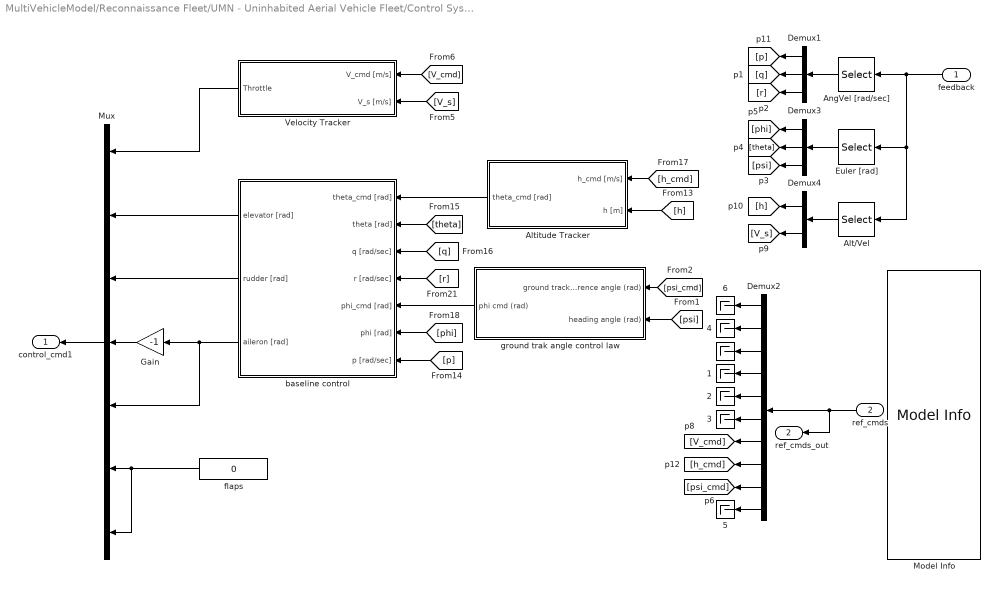
== system MultiVehicleModel/Reconnaissance Fleet/UMN - Uninhabited Aerial Vehicle Fleet/Control System/Control_Algorithm  ==
  feedback : Inport
  ref_cmds : Inport  Port=2
   {,1..6} (7 alike) : Terminator
  Alt/Vel : Selector  InputPortWidth=19  Indices=[10:11]
  Altitude Tracker : Subsystem
  AngVel [rad/sec] : Selector  InputPortWidth=19  Indices=[4:6]
  Demux1 : Demux  Outputs=3
  Demux2 : Demux  Outputs=[1 1 1 1 1 1 1 1 1 3]
  Demux3 : Demux  Outputs=3
  Demux4 : Demux  Outputs=2
  Euler [rad] : Selector  InputPortWidth=19  Indices=[1:3]
  Gain : Gain  Gain=-1
  Model Info : simulink/Model-Wide Utilities/Model Info  InitialBlockCM=None  Frame=on  DisplayStringWithTags=|  HorizontalTextAlignment=Center  LeftAlignmentValue=0.5  SourceBlockDiagram=MultiVehicleModel  TagMaxNumber=20
      | Ref Cmd Port Info
      | 
      | 1. phi_cmd
      | 2. theta_cmd
      | 3. psi_cmd
      | 4. p_cmd
      | 5. q_cmd
      | 6. r_cmd
      | 7. V_s_cmd
      | 8. h_cmd
      | 9. gndtrk_cmd
      | 10. aoa_cmd
      | 11. aos_cmd
      | 12. gamma_cmd
      | 13. signal_0
      | 14. signal_1
      | 15. signal_2
      | 16. signal_3
      | 17. signal_4
      | 18. signal_5
      | 19. signal_6
      | 20. signal_7
      | 21. signal_8
      | 22. signal_9
  Mux : Mux  Inputs=7
  Velocity Tracker : Subsystem
  baseline control : Subsystem  mask(Baseline Controller){pitch_gains=control.pitch_gains, roll_gains=control.roll_gains, yaw_damper_num=control.yaw_damper_num, yaw_damper_den=control.yaw_damper_den}
      mask prompts: pitch_gains "Pitch gains:"; roll_gains "Roll gains:"; yaw_damper_num "Yaw damper discrete transfer function numerator coefficients:"; yaw_damper_den "Yaw damper discrete transfer function denominator coefficients:"
      mask help:
      | The "Pitch gains" parameter takes a vector input in which the first term is the
      | proportional pitch tracking gain, the second term is the integral pitch
      | tracking gain, and the third term is the pitch rate proportional gain.
      |
      | The "Roll gains" parameter takes a vector input in which the first term is the
      | proportional roll tracking gain, the second term is the integral roll tracking
      | gain, and the third term is the roll rate proportional gain.
      |
      | The yaw damper parameters take vector inputs consisting of the discrete transfer
      | function numerator and denominator coefficients.
      |
      | See Mask help for a description of the control architecture.
      mask Help:
      | This is a simple baseline controller model for the Ultrastick UAVs.
      | For the pitch axis, there is a pitch damper consisting of a proportional
      | gain on the pitch rate. The output is subtracted from the output of a
      | PI control pitch angle tracker, and the result is sent to the elevator
      | command.
      | 
      | For the roll axis, there is a roll damper consisting of a proportional
      | gain (kp_RD) on the roll rate. The output is subtracted from the output of
      | a PI control roll angle tracker, and the result is sent to the aileron
      | command.
      | 
      | For the yaw axis, there is a discrete transfer function with input yawrate,
      | and output rudder.
  flaps : Constant  Value=0
  ground trak angle control law : Subsystem
  control_cmd1 : Outport
  ref_cmds_out : Outport  Port=2
  wires:
  flaps/1 -> Mux/6, Mux/7
  Mux/1 -> control_cmd1/1
  Demux3/1 -> [phi]
  feedback/1 -> AngVel [rad/sec]/1, Euler [rad]/1, Alt/Vel/1
  Demux4/1 -> [h]
  Demux4/2 -> [V_s]
  [theta] -> baseline control/2(theta [rad])
  Demux1/3 -> [r]
  Demux3/3 -> [psi]
  Gain/1 -> Mux/4
  Alt/Vel/1 -> Demux4/1
  Demux1/2 -> [q]
  Euler [rad]/1 -> Demux3/1
  AngVel [rad/sec]/1 -> Demux1/1
  Demux1/1 -> [p]
  Demux3/2 -> [theta]
  Demux2/5 -> " 2"/1
  Velocity Tracker/1("Throttle ") -> Mux/1
  Altitude Tracker/1(theta_cmd [rad]) -> baseline control/1(theta_cmd [rad])
  Demux2/6 -> " 3"/1
  Demux2/8 -> [h_cmd]
  [V_s] -> Velocity Tracker/2(V_s [m/s])
  ground trak angle control law/1(phi cmd (rad)) -> baseline control/5(phi_cmd [rad])
  [h] -> Altitude Tracker/2(h [m])
  baseline control/3(aileron [rad]) -> Gain/1, Mux/5
  baseline control/2(rudder [rad]) -> Mux/3
  baseline control/1(elevator [rad]) -> Mux/2
  ref_cmds/1 -> ref_cmds_out/1, Demux2/1
  Demux2/2 -> " 4"/1
  Demux2/9 -> [psi_cmd]
  [V_cmd] -> Velocity Tracker/1(V_cmd [m/s])
  [r] -> baseline control/4(r [rad/sec])
  [q] -> baseline control/3(q [rad/sec])
  Demux2/3 -> " "/1
  Demux2/4 -> " 1"/1
  Demux2/7 -> [V_cmd]
  [p] -> baseline control/7(p [rad/sec])
  [psi_cmd] -> ground trak angle control law/1(ground track reference angle (rad))
  Demux2/10 -> " 5"/1
  Demux2/1 -> " 6"/1
  [h_cmd] -> Altitude Tracker/1(h_cmd [m/s])
  [phi] -> baseline control/6(phi [rad])
  [psi] -> ground trak angle control law/2(heading angle (rad))

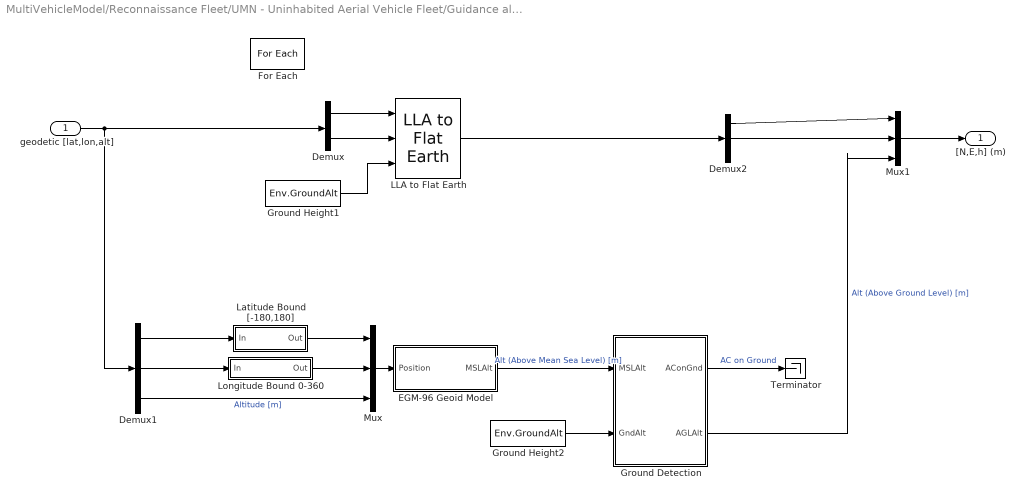
== system MultiVehicleModel/Reconnaissance Fleet/UMN - Uninhabited Aerial Vehicle Fleet/Guidance algorithm/From geodetic to NED coordinate representation ==
  geodetic [lat,lon,alt] : Inport  Partition=on  PartitionDimension=2  PartitionWidth=1
  Demux : Demux  Outputs=[2 1]
  Demux1 : Demux  Outputs=3
  Demux2 : Demux  Outputs=3
  EGM-96 Geoid Model : Subsystem  mask(EGM-96 geoid undulation model){}
      mask help: Computes the MSL (mean sea level) altitude as a function of position.
      mask init:
      | load('egm96');
      mask Help:
      | The block computes the mean-sea-level altitude relative to the WGS-84 geoid.
      | <P><B>Inputs:</B>
      | <LI>Position = the 3x1 vector of aircraft location [Latitude Longitude Altitude], in [rad rad m]</LI>
      | </P>
      | <P><B>Output:</B>
      | <LI>MSLAlt = the mean-sea-level altitude, in m</LI>
      | </P>
  For Each : ForEach  DisableCoverage=on  IndexMode=One-based
  Ground Detection : Subsystem  mask(Ground detection){}
      mask help: Computes altitude above ground and sets a flag if AGL is negative.
      mask Help:
      | The block computes the altitude above ground (AGL) and sets a flag if the AGL is negative (used for ground contact detection).
      | <P><B>Inputs:</B>
      | <LI>MSLAlt = the altitude measured from mean-sea-level, in meters</LI>
      | <LI>GndAlt = the altitude of the terrain (above MSL) at current location, in meters</LI>
      | </P>
      | <P><B>Output:</B>
      | <LI>AConGnd = the aircraft-on-ground flag (0 if aircraft above ground, 1 if aircraft on the ground)</LI>
      | <LI>AGLAlt = the altitude of the aircraft above ground</LI>
      | </P>
  Ground Height1 : Constant  Value=Env.GroundAlt
  Ground Height2 : Constant  Value=Env.GroundAlt
  LLA to Flat Earth : aerolibtransform2/LLA to Flat Earth  units=Metric (MKS)  ptype=Earth (WGS84)  F=1/298.257223563  R=6378137  LL0=FWFleet.IC.geodetic(1:2)  psi=0
  Latitude Bound [-180,180] : Subsystem
  Longitude Bound 0-360 : Subsystem  mask(Longitude bound){}
      mask help: Bounds the longitude to [0, 2pi]. When 0 bound is exceeded the longitude wraps back to 2pi; when the 2pi bound is exceeded the longitude wraps back to 0.
  Mux : Mux  Inputs=3
  Mux1 : Mux  Inputs=3
  Terminator : Terminator
  "[N,E,h] (m)" : Outport  ConcatenationDimension=2
  wires:
  Demux/1 -> LLA to Flat Earth/1
  Demux/2 -> LLA to Flat Earth/2
  geodetic [lat,lon,alt]/1 -> Demux/1, Demux1/1
  Ground Height1/1 -> LLA to Flat Earth/3
  Demux1/3 -> Mux/3  "Altitude [m]"
  Ground Height2/1 -> Ground Detection/2(GndAlt)
  EGM-96 Geoid Model/1(MSLAlt) -> Ground Detection/1(MSLAlt)  "Alt (Above Mean Sea Level) [m]"
  Mux/1 -> EGM-96 Geoid Model/1(Position)
  Longitude Bound 0-360/1(Out) -> Mux/2
  Latitude Bound [-180,180]/1(Out) -> Mux/1
  Demux1/2 -> Longitude Bound 0-360/1(In)
  Demux1/1 -> Latitude Bound [-180,180]/1(In)
  Ground Detection/1(AConGnd) -> Terminator/1  "AC on Ground"
  Ground Detection/2(AGLAlt) -> Mux1/3  "Alt (Above Ground Level) [m]"
  LLA to Flat Earth/1 -> Demux2/1
  Demux2/1 -> Mux1/1
  Demux2/2 -> Mux1/2
  Mux1/1 -> "[N,E,h] (m)"/1

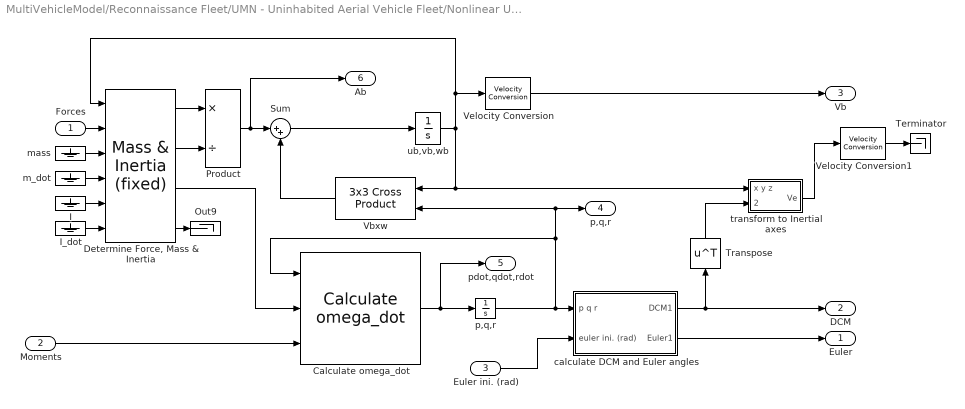
== system MultiVehicleModel/Reconnaissance Fleet/UMN - Uninhabited Aerial Vehicle Fleet/Nonlinear UAV Model/6DoF EOM ==
  Forces : Inport
  Moments : Inport  Port=2
  Euler ini. (rad) : Inport  Port=3
  Calculate omega_dot : aerolib6dofsys/Calculate omega_dot  SystemSampleTime=-1
  "Determine Force, Mass & Inertia" : aerolib6dofsys/Mass & Inertia (fixed)  SystemSampleTime=-1
  I : Ground
  I_dot : Ground
  Out9 : Terminator
  Product : Product  Inputs=*/  SaturateOnIntegerOverflow=on  OutDataTypeStr=Inherit: Same as first input
  Sum : Sum  Inputs=|++  SaturateOnIntegerOverflow=on
  Terminator : Terminator
  Transpose : Math  Operator=transpose  SaturateOnIntegerOverflow=on
  Vbxw : aerolibutil/3x3 Cross Product
  Velocity Conversion : aerolibconvert2/Velocity Conversion  IU=m/s  OU=m/s
  Velocity Conversion1 : aerolibconvert2/Velocity Conversion  IU=m/s  OU=m/s
  calculate DCM and Euler angles : Subsystem
  m_dot : Ground
  mass : Ground
  "p,q,r " : Integrator  InitialCondition=pm_0
  "transform to Inertial axes " : Subsystem  mask(Vector Transformation){}
      mask Display: disp('L_EB')
  ub,vb,wb : Integrator  InitialCondition=convvel(Vm_0,'m/s','m/s')
  Euler : Outport
  DCM : Outport  Port=2
  Vb : Outport  Port=3
  p,q,r : Outport  Port=4
  pdot,qdot,rdot : Outport  Port=5
  Ab : Outport  Port=6
  wires:
  Velocity Conversion1/1 -> Terminator/1
  Velocity Conversion/1 -> Vb/1
  "Determine Force, Mass & Inertia"/3 -> Calculate omega_dot/2
  calculate DCM and Euler angles/2(Euler1) -> Euler/1
  Vbxw/1 -> Sum/2
  ub,vb,wb/1 -> Velocity Conversion/1, "Determine Force, Mass & Inertia"/1, "transform to Inertial axes "/1(x y z), Vbxw/1
  Sum/1 -> ub,vb,wb/1
  "transform to Inertial axes "/1(Ve) -> Velocity Conversion1/1
  "p,q,r "/1 -> Calculate omega_dot/1, p,q,r/1, Vbxw/2, calculate DCM and Euler angles/1("p q r ")
  Moments/1 -> Calculate omega_dot/3
  Forces/1 -> "Determine Force, Mass & Inertia"/2
  Product/1 -> Sum/1, Ab/1
  calculate DCM and Euler angles/1(DCM1) -> Transpose/1, DCM/1
  Transpose/1 -> "transform to Inertial axes "/2(transform coefficients)
  mass/1 -> "Determine Force, Mass & Inertia"/3
  "Determine Force, Mass & Inertia"/2 -> Product/2
  m_dot/1 -> "Determine Force, Mass & Inertia"/4
  "Determine Force, Mass & Inertia"/4 -> Out9/1
  Calculate omega_dot/1 -> pdot,qdot,rdot/1, "p,q,r "/1
  I/1 -> "Determine Force, Mass & Inertia"/5
  I_dot/1 -> "Determine Force, Mass & Inertia"/6
  "Determine Force, Mass & Inertia"/1 -> Product/1
  Euler ini. (rad)/1 -> calculate DCM and Euler angles/2(euler ini. (rad))

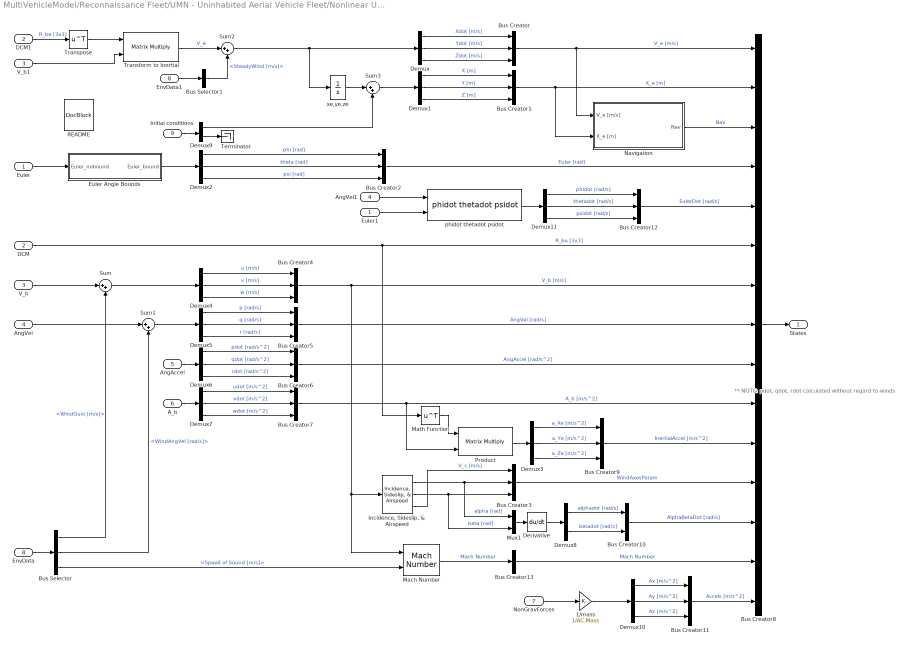
== system MultiVehicleModel/Reconnaissance Fleet/UMN - Uninhabited Aerial Vehicle Fleet/Nonlinear UAV Model/Auxiliary Equations ==
  note: ** NOTE: pdot, qdot, rdot calculated without regard to winds
  Euler : Inport
  DCM : Inport  Port=2
  V_b : Inport  Port=3
  AngVel : Inport  Port=4
  AngAccel : Inport  Port=5
  A_b : Inport  Port=6
  NonGravForces : Inport  Port=7
  EnvData : Inport  Port=8
  Initial conditions : Inport  Port=9
  1/mass : Gain  Gain=1/AC.Mass
  AngVel1 : InportShadow  Port=4
  Bus Creator{,1..7,9,11..12} (11 alike) : BusCreator  Inputs=3
  Bus Creator10 : BusCreator  Inputs=2
  Bus Creator13 : BusCreator  Inputs=1
  Bus Creator8 : BusCreator  Inputs=15
  Bus Selector : BusSelector  OutputSignals=WindGust [m/s],WindAngVel [rad/s],Speed of Sound [m/s]
  Bus Selector1 : BusSelector  OutputSignals=SteadyWind [m/s]
  DCM1 : InportShadow  Port=2
  Demux{,1..7,10..11} (10 alike) : Demux  Outputs=3
  Demux8 : Demux  Outputs=2
  Demux9 : Demux  Outputs=[3 1]
  Derivative : Derivative
  EnvData1 : InportShadow  Port=8
  Euler Angle Bounds : Subsystem
  Euler1 : InportShadow
  "Incidence, Sideslip, & Airspeed" : aerolibasang/Incidence, Sideslip, & Airspeed
  Mach Number : aerolibasang/Mach Number
  Math Function : Math  Operator=transpose  SaturateOnIntegerOverflow=on
  Mux1 : Mux  Inputs=2
  Navigation : Subsystem  Description=|
      | This model produces the followng navigation data for the UAV flight:
      |                                                                     
      | * Geodetic Latitude                                                 
      | * Geodetic Longitude                                                
      | * Geodetic Altitude                                                 
      | * Altitude above Mean Sea Level                                     
      | * Gravitational acceleration vector
  Product : Product  Multiplication=Matrix(*)  RndMeth=Zero
  README : simulink/Model-Wide Utilities/DocBlock  DocumentType=Text
      content=|
      | Auxiliary Equations
      |
      | This block computes other relevant variables (such as angle of attack,
      | indicated airspeed, etc) from state data. Part of this block is simply to
      | assign signals name and create the States bus.
      |
      | Working from the top of the block downwards:
      |
      | The inertial velocity, V_e, is computed by using the Direction Cosine
      | Matrix (DCM) to transform the body-axis velocities (u,v,w) to the
      | inertial frame. The steady state winds are then added, and the result is
      | V_e. This is integrated to obtain the inertial position, X_e.  The
      | initial condition of the X_e integrator is set by
      | TrimCondition.InertialIni. V_e and X_e are inputs to the Navigation
      | block- see that blocks README for details.
      |
      | Euler angles are bounded by +\- [pi/2, pi, 2*pi] respectively. The time
      | derivatives of the Euler angles are computed using the body-axis rates
      | and the Euler angles.
      |
      | The DCM is included in the States bus as "R_be [3x3]".
      |
      | Body axis velocites and rates, and their derivatives are included. The
      | unsteady (turbulence and gusts) winds are added to the body axis
      | velocities and rates.
      |
      | Inertial accelerations are computed by transforming the body-axis
      | accelerations with the DCM. This step is simplified since we are using a
      | non-rotating Earth.
      |
      | WindAxesParam is the true airspeed, angle of attack, and sideslip angle.
      | The derivatives of alpha and beta are computed using a deriative block.
      | Mach number is simply the ratio between true airspeed and the speed of
      | sound.
      |
      | Accels [m/s^2] is what an accelerometer would read onboard the aircraft.
      |
      | *Note on winds: dividing the wind components into steady and unsteady
      | components is necessary because we do not use an intermediate atmospheric
      | reference frame to account for the motion of the air mass relative to the
      | Earth. We can approximate the physical effects of wind without an
      | additional reference frame by splitting the wind into steady and unsteady
      | components, where the steady component is added to the inertial
      | velocities and the unsteady component is added to the body-axis
      | velocities allows us to
  Sum{,1..3} (4 alike) : Sum  Inputs=|++
  Terminator : Terminator
  Transform to Inertial : Product  Multiplication=Matrix(*)  RndMeth=Zero
  Transpose : Math  Operator=transpose  SaturateOnIntegerOverflow=on
  V_b1 : InportShadow  Port=3
  phidot thetadot psidot : aerolib6dofsys/DCM & Euler Angles (Euler)/phidot thetadot psidot
  xe,ye,ze : Integrator  InitialCondition=[0;0;0]
  States : Outport
  wires:
  Mach Number/1 -> Bus Creator13/1  "Mach Number"
  Demux8/2 -> Bus Creator10/2  "betadot [rad/s]"
  Demux8/1 -> Bus Creator10/1  "alphadot [rad/s]"
  Bus Creator10/1 -> Bus Creator8/13  "AlphaBetaDot [rad/s]"
  Derivative/1 -> Demux8/1
  Mux1/1 -> Derivative/1
  "Incidence, Sideslip, & Airspeed"/3 -> Bus Creator3/1  "V_s [m/s]"
  "Incidence, Sideslip, & Airspeed"/2 -> Mux1/2, Bus Creator3/3  "beta [rad]"
  "Incidence, Sideslip, & Airspeed"/1 -> Mux1/1, Bus Creator3/2  "alpha [rad]"
  Bus Creator8/1 -> States/1
  Navigation/1(Nav) -> Bus Creator8/3  "Nav"
  Bus Creator11/1 -> Bus Creator8/15  "Accels [m/s^2]"
  Euler1/1 -> phidot thetadot psidot/2
  AngVel1/1 -> phidot thetadot psidot/1
  Bus Selector/1 -> Sum/2  "<WindGust [m/s]>"
  Bus Selector/2 -> Sum1/2  "<WindAngVel [rad/s]>"
  Bus Creator9/1 -> Bus Creator8/11  "InertialAccel [m/s^2]"
  Demux3/2 -> Bus Creator9/2  "a_Ye [m/s^2]"
  Demux3/3 -> Bus Creator9/3  "a_Ze [m/s^2]"
  Demux3/1 -> Bus Creator9/1  "a_Xe [m/s^2]"
  Product/1 -> Demux3/1
  Math Function/1 -> Product/1
  V_b/1 -> Sum/1
  AngVel/1 -> Sum1/1
  Sum/1 -> Demux4/1
  Sum1/1 -> Demux5/1
  Bus Selector/3 -> Mach Number/2  "<Speed of Sound [m/s]>"
  EnvData/1 -> Bus Selector/1
  Bus Creator13/1 -> Bus Creator8/14  "Mach Number"
  Bus Creator3/1 -> Bus Creator8/12  "WindAxesParam"
  A_b/1 -> Demux7/1
  Demux7/3 -> Bus Creator7/3  "wdot [m/s^2]"
  Demux7/2 -> Bus Creator7/2  "vdot [m/s^2]"
  Demux7/1 -> Bus Creator7/1  "udot [m/s^2]"
  Bus Creator7/1 -> Bus Creator8/10, Product/2  "A_b [m/s^2]"
  AngAccel/1 -> Demux6/1
  Demux6/3 -> Bus Creator6/3  "rdot [rad/s^2]"
  Demux6/2 -> Bus Creator6/2  "qdot [rad/s^2]"
  Demux6/1 -> Bus Creator6/1  "pdot [rad/s^2]"
  Bus Creator6/1 -> Bus Creator8/9  "AngAccel [rad/s^2]"
  Demux5/3 -> Bus Creator5/3  "r [rad/s]"
  Demux5/2 -> Bus Creator5/2  "q [rad/s]"
  Demux5/1 -> Bus Creator5/1  "p [rad/s]"
  Bus Creator5/1 -> Bus Creator8/8  "AngVel [rad/s]"
  Demux4/3 -> Bus Creator4/3  "w [m/s]"
  Demux4/2 -> Bus Creator4/2  "v [m/s]"
  Demux4/1 -> Bus Creator4/1  "u [m/s]"
  Bus Creator4/1 -> Mach Number/1, "Incidence, Sideslip, & Airspeed"/1, Bus Creator8/7  "V_b [m/s]"
  DCM/1 -> Bus Creator8/6, Math Function/1  "R_be [3x3]"
  Demux2/2 -> Bus Creator2/2  "theta [rad]"
  Demux2/1 -> Bus Creator2/1  "phi [rad]"
  Bus Creator2/1 -> Bus Creator8/4  "Euler [rad]"
  Demux1/3 -> Bus Creator1/3  "Z [m]"
  Demux1/2 -> Bus Creator1/2  "Y [m]"
  Demux1/1 -> Bus Creator1/1  "X [m]"
  Bus Creator1/1 -> Bus Creator8/2, Navigation/2(X_e [m])  "X_e [m]"
  Demux/3 -> Bus Creator/3  "Zdot [m/s]"
  Demux/2 -> Bus Creator/2  "Ydot [m/s]"
  Demux/1 -> Bus Creator/1  "Xdot [m/s]"
  Bus Creator/1 -> Bus Creator8/1, Navigation/1(V_e [m/s])  "V_e [m/s]"
  NonGravForces/1 -> 1/mass/1
  1/mass/1 -> Demux10/1
  Demux10/1 -> Bus Creator11/1  "Ax [m/s^2]"
  Demux10/2 -> Bus Creator11/2  "Ay [m/s^2]"
  Demux10/3 -> Bus Creator11/3  "Az [m/s^2]"
  Demux11/3 -> Bus Creator12/3  "psidot [rad/s]"
  Demux11/2 -> Bus Creator12/2  "thetadot [rad/s]"
  Demux11/1 -> Bus Creator12/1  "phidot [rad/s]"
  Bus Creator12/1 -> Bus Creator8/5  "EulerDot [rad/s]"
  phidot thetadot psidot/1 -> Demux11/1
  Transpose/1 -> Transform to Inertial/1
  DCM1/1 -> Transpose/1  "R_be [3x3]"
  EnvData1/1 -> Bus Selector1/1
  Transform to Inertial/1 -> Sum2/1  "V_e"
  Bus Selector1/1 -> Sum2/2  "<SteadyWind [m/s]>"
  Sum2/1 -> Demux/1, xe,ye,ze/1
  V_b1/1 -> Transform to Inertial/2
  Euler/1 -> Euler Angle Bounds/1(Euler_nobound)
  Euler Angle Bounds/1(Euler_bound) -> Demux2/1
  Sum3/1 -> Demux1/1
  xe,ye,ze/1 -> Sum3/1
  Initial conditions/1 -> Demux9/1
  Demux9/1 -> Sum3/2
  Demux2/3 -> Bus Creator2/3  "psi [rad]"
  Demux9/2 -> Terminator/1
